simulink model "gesture_sim"  (R2022b)
settings: Solver=VariableStepAuto  StartTime=0.0  StopTime=10.0  RelTol=1e-3
settings Model: Creator=Timi Banjo  LastModifiedBy=Timi Banjo

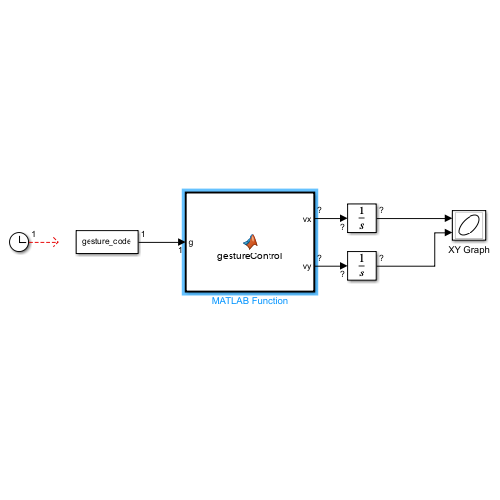
[thumbnail: Simulink's stored preview of the top-level diagram]
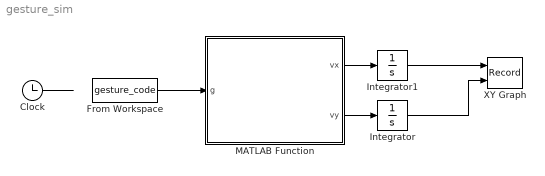
== system gesture_sim ==
  Clock : Clock
  From Workspace : FromWorkspace  VariableName=gesture_code
  Integrator : Integrator
  Integrator1 : Integrator
  MATLAB Function : MATLAB Function  TreatAsAtomicUnit=on
  XY Graph : Record  FileSettingsInternal="{\"entries\":[{\"content\":{\"excelSettings\":{\"content\":{},\"type\":\"Streamout.ExcelSettings\"}},\"type\":\"Streamout.FileSettingStorage\",\"uuid\":\"c3bd502a-33b7-408e-8752-6e9ddd59f2c3\"}],\"packageUris\":[\"http://schema.mathworks.com/mf0/streamout_blocks/R2020a\"],\"version\":\"1.0\"}"  Layout=[1 1]  SignalsInternal="{\"entries\":[{\"content\":{\"signals\":[{\"content\":{\"blockPath\":[\"gesture_sim/XY Graph\"],\"channel\":[],\"dimensions\":[1],\"domain\":\"gesture_sim/XY Graph\",\"lineColor\":\"#a2142f\",\"plots\":[],\"port\":1,\"sid\":[\"\"],\"signalID\":529,\"signalName\":\"Integrator1\"},\"type\":\"RecordBlkView.Signal\",\"uuid\":\"5e397726-2fb4-4190-97af-135726741134\"},{\"content\":{\"blockPath\":[\"gesture_sim/XY Graph\"],\"channel\":[],\"dimensions\":[1],\"domain\":\"gesture_sim/XY Graph\",\"lineColor\":\"#139fff\",\"plots\":[],\"port\":2,\"sid\":[\"\"],\"signalID\":533,\"signalName\":\"Integrator\"},\"type\":\"RecordBlkView.Signal\",\"uuid\":\"b4babfd1-02ac-4ea5-9af1-fe42faddf626\"}]},\"type\":\"RecordBlkView.InputSignals\",\"uuid\":\"61d77186-72fb-41af-86c4-0d4c0a7b6c0b\"}],\"packageUris\":[\"http://schema.mathworks.com/mf0/streamout_blocks/R2020a\"],\"version\":\"1.0\"}"  VisualizationBindings="{\"xyplotplugin\":{\"info\":[{\"series\":[],\"subplotID\":1}]}}"  CompatibilityTag=XY
  wires:
  From Workspace/1 -> MATLAB Function/1(g)
  MATLAB Function/1(vx) -> Integrator1/1
  MATLAB Function/2(vy) -> Integrator/1
  Integrator/1 -> XY Graph/2
  Clock/1 -> ?
  Integrator1/1 -> XY Graph/1

== matlab function gesture_sim/MATLAB Function ==
  data: g input; vx output; vy output
function [vx, vy] = gestureControl(g)
% g = gesture code
vx = 0; vy = 0;
switch g
    case 1  % forward
        vy = 1;
    case 2  % backward
        vy = -1;
    case 3  % left
        vx = -1;
    case 4  % right
        vx = 1;
    case 5  % stop
        vx = 0;
        vy = 0;

classdef app1 < matlab.apps.AppBase

    % Properties that correspond to app components
    properties (Access = public)
        UIFigure  matlab.ui.Figure
        qButton   matlab.ui.control.Button
        xButton   matlab.ui.control.Button
        dButton   matlab.ui.control.Button
        aButton   matlab.ui.control.Button
        sButton   matlab.ui.control.Button
        wButton   matlab.ui.control.Button
    end

    
    properties (Access = private)
        GestureCode = 0; % 0 = no command
 % Description
        
    GestureTimer % This is the timer object that runs in the background
 % Description
    end
    

    % Callbacks that handle component events
    methods (Access = private)

        % Code that executes after component creation
        function startupFcn(app)

    % Create and start a timer to update gesture_code in the workspace
    app.GestureTimer = timer( ...
        'ExecutionMode', 'fixedRate', ... % It runs repeatedly
        'Period', 0.1, ...                % Every 0.1 seconds
        'TimerFcn', @(~,~) updateGestureCode(app));
 % Send GestureCode to workspace
     % Store gesture code as a time series in the base workspace
    function updateGestureCode(app)
        persistent t;
        persistent data;

        if isempty(t)
            t = 0;
            data = [];
        else
            t = t + 0.1; % time step
        end

        data = [data; t, app.GestureCode];
        assignin('base', 'gesture_code', data);
    end


    start(app.GestureTimer); % Start the timer

        end

        % Button pushed function: wButton
        function wButtonPushed(app, event)
            function ForwardButtonPushed(app, event)
    app.GestureCode = 1; % 1 = forward
end
        end

        % Button pushed function: sButton
        function sButtonPushed(app, event)
            function BackwardButtonPushed(app, event)
    app.GestureCode = 2; % 2 = backward
end
        end

        % Button pushed function: aButton
        function aButtonPushed(app, event)
            function LeftButtonPushed(app, event)
    app.GestureCode = 3; % 3 = left
end
        end

        % Button pushed function: dButton
        function dButtonPushed(app, event)
            function RightButtonPushed(app, event)
    app.GestureCode = 4; % 4 = right
end
        end

        % Button pushed function: xButton
        function xButtonPushed(app, event)
            function StopButtonPushed(app, event)
    app.GestureCode = 5; % 5 = stop
end
        end

        % Close request function: UIFigure
        function UIFigureCloseRequest(app, event)
            delete(app)
            function CloseRequestFcn(app, event)
    % Stop and delete the timer when app closes
    if ~isempty(app.GestureTimer)
        stop(app.GestureTimer);
        delete(app.GestureTimer);
    end

    delete(app); % Close the app properly
end

        end
    end

    % Component initialization
    methods (Access = private)

        % Create UIFigure and components
        function createComponents(app)

            % Create UIFigure and hide until all components are created
            app.UIFigure = uifigure('Visible', 'off');
            app.UIFigure.Position = [100 100 640 480];
            app.UIFigure.Name = 'MATLAB App';
            app.UIFigure.CloseRequestFcn = createCallbackFcn(app, @UIFigureCloseRequest, true);

            % Create wButton
            app.wButton = uibutton(app.UIFigure, 'push');
            app.wButton.ButtonPushedFcn = createCallbackFcn(app, @wButtonPushed, true);
            app.wButton.Position = [95 337 100 23];
            app.wButton.Text = 'w';

            % Create sButton
            app.sButton = uibutton(app.UIFigure, 'push');
            app.sButton.ButtonPushedFcn = createCallbackFcn(app, @sButtonPushed, true);
            app.sButton.Position = [95 296 100 23];
            app.sButton.Text = 's';

            % Create aButton
            app.aButton = uibutton(app.UIFigure, 'push');
            app.aButton.ButtonPushedFcn = createCallbackFcn(app, @aButtonPushed, true);
            app.aButton.Position = [95 257 100 23];
            app.aButton.Text = 'a';

            % Create dButton
            app.dButton = uibutton(app.UIFigure, 'push');
            app.dButton.ButtonPushedFcn = createCallbackFcn(app, @dButtonPushed, true);
            app.dButton.Position = [251 336 100 23];
            app.dButton.Text = 'd';

            % Create xButton
            app.xButton = uibutton(app.UIFigure, 'push');
            app.xButton.ButtonPushedFcn = createCallbackFcn(app, @xButtonPushed, true);
            app.xButton.Position = [251 296 100 23];
            app.xButton.Text = 'x';

            % Create qButton
            app.qButton = uibutton(app.UIFigure, 'push');
            app.qButton.Position = [251 256 100 23];
            app.qButton.Text = 'q';

            % Show the figure after all components are created
            app.UIFigure.Visible = 'on';
        end
    end

    % App creation and deletion
    methods (Access = public)

        % Construct app
        function app = app1

            % Create UIFigure and components
            createComponents(app)

            % Register the app with App Designer
            registerApp(app, app.UIFigure)

            % Execute the startup function
            runStartupFcn(app, @startupFcn)

            if nargout == 0
                clear app
            end
        end

        % Code that executes before app deletion
        function delete(app)

            % Delete UIFigure when app is deleted
            delete(app.UIFigure)
        end
    end
end
end
